simulink model "Systeme_a_Optimse"  (R2023a)
settings: Solver=ode45  StartTime=0.0  StopTime=5000  RelTol=1e-3  EnableMultiTasking=on
values from neighbouring files (symbols this model uses):
  Kd = abs(xx(3))    [PSO.m]    (also in tracklsq.m = abs(pid(3)))
  Ki = abs(xx(2))    [PSO.m]    (also in tracklsq.m = abs(pid(2)))
  Kp = abs(xx(1))    [PSO.m]    (also in tracklsq.m = abs(pid(1)))
settings Model: Creator=zina  LastModifiedBy=mluser
settings SolverCC: AlgebraicLoopSolver=TrustRegion
settings DataIOCC: LimitDataPoints=on  SaveFormat=Array  ReturnWorkspaceOutputs=off
settings OptimizationCC: LifeSpan=inf
settings DebuggingCC: SolverPrmCheckMsg=warning  UnconnectedInputMsg=warning  UnconnectedOutputMsg=warning  UnconnectedLineMsg=warning  SFUnexpectedBacktrackingDiag=warning  SFNoUnconditionalDefaultTransitionDiag=warning  SFExecutionAtInitializationDiag=none  ArithmeticOperatorsInVariantConditions=warning
settings HardwareCC: ProdBitPerPointer=32  ProdBitPerSizeT=32  ProdBitPerPtrDiffT=32  ProdLargestAtomicFloat=None  ProdIntDivRoundTo=Undefined  ProdEndianess=Unspecified  ProdWordSize=32  ProdHWDeviceType=32-bit Generic
settings ModelReferenceCC: PropagateSignalLabelsOutOfModel=off
settings SFSimCC: SimUseLocalCustomCode=off  CustomCodeUndefinedFunction=UseInterfaceOnly
settings RTWCC: RTWUseLocalCustomCode=off
settings CodeAppCC: StateflowObjectComments=on
settings GRTTargetCC: TargetLangStandard=C89/C90 (ANSI)
settings ConfigComp: CovMetricSettings=dw  CovSaveCumulativeToWorkspaceVar=on  CovSaveSingleToWorkspaceVar=on  CovExternalEMLEnable=off  CovSFcnEnable=off

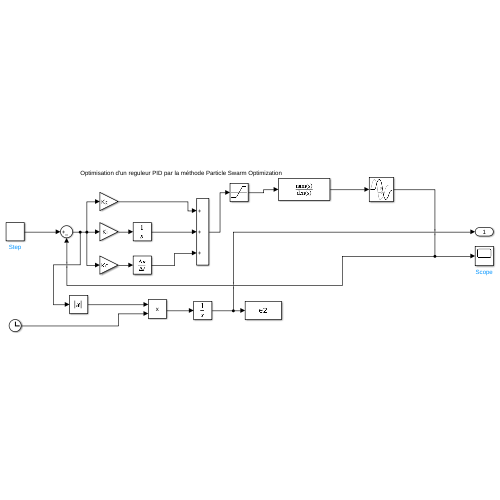
[thumbnail: Simulink's stored preview of the top-level diagram]
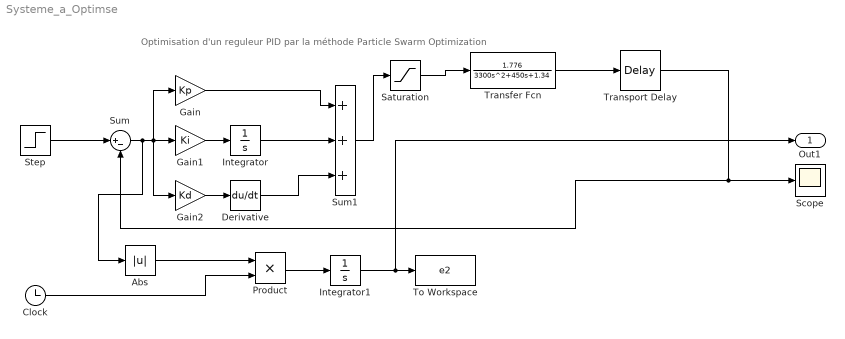
== system Systeme_a_Optimse ==
  note: Optimisation d'un reguleur PID par la méthode Particle Swarm Optimization
  Abs : Abs  SaturateOnIntegerOverflow=off
  Clock : Clock
  Derivative : Derivative
  Gain : Gain  Gain=Kp
  Gain1 : Gain  Gain=Ki
  Gain2 : Gain  Gain=Kd
  Integrator : Integrator
  Integrator1 : Integrator
  Product : Product
  Saturation : Saturate
  Scope : Scope
  Step : Step  SampleTime=0
  Sum : Sum  Inputs=|+-
  Sum1 : Sum  Inputs=+++
  To Workspace : ToWorkspace  VariableName=e2  SampleTime=-1
      settings: MaxDataPoints=1
  Transfer Fcn : TransferFcn  Numerator=[1.776]  Denominator=[3300 450 1.34]
  Transport Delay : TransportDelay
  Out1 : Outport
  wires:
  Integrator/1 -> Sum1/2
  Gain/1 -> Sum1/1
  Gain1/1 -> Integrator/1
  Derivative/1 -> Sum1/3
  Gain2/1 -> Derivative/1
  Sum/1 -> Abs/1, Gain2/1, Gain1/1, Gain/1
  Step/1 -> Sum/1
  Product/1 -> Integrator1/1
  Integrator1/1 -> Out1/1, To Workspace/1
  Abs/1 -> Product/1
  Clock/1 -> Product/2
  Sum1/1 -> Saturation/1
  Saturation/1 -> Transfer Fcn/1
  Transfer Fcn/1 -> Transport Delay/1
  Transport Delay/1 -> Sum/2, Scope/1
